simulink model "MassSpringDamperInSimulink"  (R2024a)
settings: Solver=VariableStepAuto  StartTime=0.0  StopTime=10.0  RelTol=1e-3
undefined symbols (not defined in the file): b, k, m

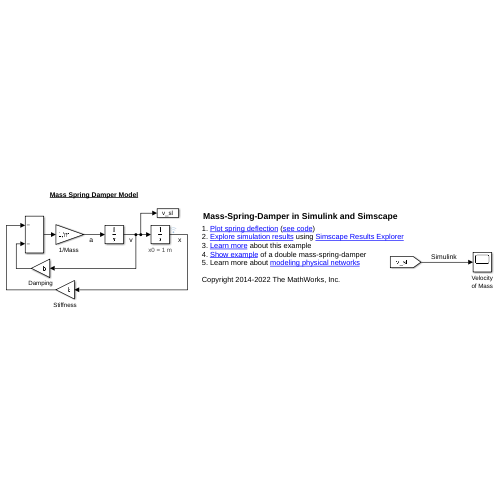
[thumbnail: Simulink's stored preview of the top-level diagram]
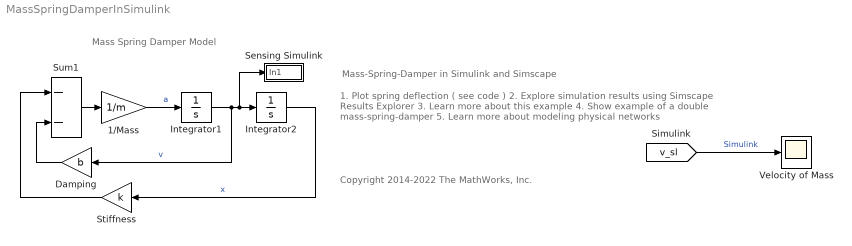
== system MassSpringDamperInSimulink ==
  note: Mass Spring Damper Model
  note: Copyright 2014-2022 The MathWorks, Inc.
  note: 1. Plot spring deflection ( see code )
      | 2. Explore simulation results using Simscape Results Explorer
      | 3. Learn more about this example
      | 4. Show example of a double mass-spring-damper
      | 5. Learn more about modeling physical networks
  note: Mass-Spring-Damper in Simulink and Simscape
  "1/Mass " : Gain  Gain=1/m  SaturateOnIntegerOverflow=on  OutDataTypeStr=Inherit: Same as input  ParamDataTypeStr=Inherit: Same as input
  Damping : Gain  Gain=b  SaturateOnIntegerOverflow=on  OutDataTypeStr=Inherit: Same as input  ParamDataTypeStr=Inherit: Same as input
  Integrator1 : Integrator
  Integrator2 : Integrator  InitialCondition=1
      settings: AttributesFormatString=x0 = %<InitialCondition> m
  Sensing Simulink : Subsystem
      mask Display: disp('v_sl')
  Stiffness : Gain  Gain=k  SaturateOnIntegerOverflow=on  OutDataTypeStr=Inherit: Same as input  ParamDataTypeStr=Inherit: Same as input
  Sum1 : Sum  Inputs=--  InputSameDT=on  SaturateOnIntegerOverflow=on  OutDataTypeStr=Inherit: Same as first input
  Velocity of Mass : Scope
  wires:
  Damping/1 -> Sum1/2
  Stiffness/1 -> Sum1/1
  Integrator1/1 -> Sensing Simulink/1(In1), Integrator2/1, Damping/1  "v"
  Integrator2/1 -> Stiffness/1  "x"
  "1/Mass "/1 -> Integrator1/1  "a"
  Sum1/1 -> "1/Mass "/1
  [v_sl] -> Velocity of Mass/1  "Simulink"

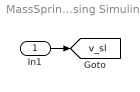
== system MassSpringDamperInSimulink/Sensing Simulink ==
  In1 : Inport
  tag scope: v_sl=global
  wires:
  In1/1 -> [v_sl]
